simulink model "G59_LKAS_Carsim"  (R2018b)
settings: Solver=FixedStepDiscrete  StartTime=0.0  StopTime=30  FixedStep=0.001  RelTol=1e-3
InitFcn:
  | %{
  | delete_block('G59_LKAS_CarSim/LL');
  | delete_block('G59_LKAS_CarSim/LLClb');
  | path=cd('D:\Work\02_LKA\LKAS');
  | getFileName=ls(strcat(pwd,'\*.slx'));
  | filename = getFileName(1:4);
  | open_system(filename);
  | add_block('LKAS/LKAS/LL','G59_LKAS_CarSim/LL');
  | add_block('LKAS/LKAS/LLClb','G59_LKAS_CarSim/LLClb');
  | close_system(filename);
  | path=cd('D:\Program Files (x86)\CarSim2019.1_Data_LKA');
  | %}
model workspace (MAT data in the model file):
  LKA_CarWidth = Simulink.Parameter
  LKA_CarWidth.Value = 1.88
  LKA_CarWidth.DataType = 'single'
  LKA_CarWidth.Dimensions = [1 1]
  LKA_SampleTime = Simulink.Parameter
  LKA_SampleTime.Value = 0.001
  LKA_SampleTime.DataType = 'single'
  LKA_SampleTime.Dimensions = [1 1]
  LKA_StrRatio_C = Simulink.Parameter
  LKA_StrRatio_C.Value = 15.3
  LKA_StrRatio_C.DataType = 'single'
  LKA_StrRatio_C.Dimensions = [1 1]
  LKA_Veh2CamL_C = Simulink.Parameter
  LKA_Veh2CamL_C.Value = 3.68
  LKA_Veh2CamL_C.DataType = 'single'
  LKA_Veh2CamL_C.Dimensions = [1 1]
  LKA_Veh2CamW_C = Simulink.Parameter
  LKA_Veh2CamW_C.Value = 0.94
  LKA_Veh2CamW_C.DataType = 'single'
  LKA_Veh2CamW_C.Dimensions = [1 1]
  LKA_WhlBaseL_C = Simulink.Parameter
  LKA_WhlBaseL_C.Value = 2.8
  LKA_WhlBaseL_C.DataType = 'single'
  LKA_WhlBaseL_C.Dimensions = [1 1]
  LL_CompSWA_C = Simulink.Parameter
  LL_CompSWA_C.Value = 0
  LL_CompSWA_C.DataType = 'single'
  LL_CompSWA_C.Dimensions = [1 1]
  LL_CrvtPrvwT_C = Simulink.Parameter
  LL_CrvtPrvwT_C.Value = 0.45
  LL_CrvtPrvwT_C.DataType = 'single'
  LL_CrvtPrvwT_C.Dimensions = [1 1]
  LL_DesDvt_C = Simulink.Parameter
  LL_DesDvt_C.Value = 0.2
  LL_DesDvt_C.DataType = 'single'
  LL_DesDvt_C.Dimensions = [1 1]
  LL_DvtComp_C = Simulink.Parameter
  LL_DvtComp_C.Value = 0
  LL_DvtComp_C.DataType = 'single'
  LL_DvtComp_C.Dimensions = [1 1]
  LL_DvtPrvwT_C = Simulink.Parameter
  LL_DvtPrvwT_C.Value = 0.45
  LL_DvtPrvwT_C.DataType = 'single'
  LL_DvtPrvwT_C.Dimensions = [1 1]
  LL_DvtSpdDet_vDvtSpdMin_C = Simulink.Parameter
  LL_DvtSpdDet_vDvtSpdMin_C.Value = 0
  LL_DvtSpdDet_vDvtSpdMin_C.DataType = 'single'
  LL_DvtSpdDet_vDvtSpdMin_C.Dimensions = [1 1]
  LL_HdAgExT_C = Simulink.Parameter
  LL_HdAgExT_C.Value = 15
  LL_HdAgExT_C.DataType = 'single'
  LL_HdAgExT_C.Dimensions = [1 1]
  LL_HdAgPrvwT_C = Simulink.Parameter
  LL_HdAgPrvwT_C.Value = 0.45
  LL_HdAgPrvwT_C.DataType = 'single'
  LL_HdAgPrvwT_C.Dimensions = [1 1]
  LL_LAccMax_C = Simulink.Parameter
  LL_LAccMax_C.Value = 3
  LL_LAccMax_C.DataType = 'single'
  LL_LAccMax_C.Dimensions = [1 1]
  LL_LAccRMax_C = Simulink.Parameter
  LL_LAccRMax_C.Value = 5
  LL_LAccRMax_C.DataType = 'single'
  LL_LAccRMax_C.Dimensions = [1 1]
  LL_LDWS_SUPPRESS_HEADING = Simulink.Parameter
  LL_LDWS_SUPPRESS_HEADING.Value = 2
  LL_LDWS_SUPPRESS_HEADING.DataType = 'single'
  LL_LDWS_SUPPRESS_HEADING.Dimensions = [1 1]
  LL_LDW_EarliestWarnLine_C = Simulink.Parameter
  LL_LDW_EarliestWarnLine_C.Value = 0.3
  LL_LDW_EarliestWarnLine_C.DataType = 'single'
  LL_LDW_EarliestWarnLine_C.Dimensions = [1 1]
  LL_LDW_LatestWarnLine_C = Simulink.Parameter
  LL_LDW_LatestWarnLine_C.Value = -0.4
  LL_LDW_LatestWarnLine_C.DataType = 'single'
  LL_LDW_LatestWarnLine_C.Dimensions = [1 1]
  LL_LFClb_TFC_FfCtlRatio_C = Simulink.Parameter
  LL_LFClb_TFC_FfCtlRatio_C.Value = 1
  LL_LFClb_TFC_FfCtlRatio_C.DataType = 'single'
  LL_LFClb_TFC_FfCtlRatio_C.Dimensions = [1 1]
  LL_LFClb_TFC_KdBalance_C = Simulink.Parameter
  LL_LFClb_TFC_KdBalance_C.Value = 0
  LL_LFClb_TFC_KdBalance_C.DataType = 'single'
  LL_LFClb_TFC_KdBalance_C.Dimensions = [1 1]
  LL_LFClb_TFC_KdMaxSWA_C = Simulink.Parameter
  LL_LFClb_TFC_KdMaxSWA_C.Value = 20
  LL_LFClb_TFC_KdMaxSWA_C.DataType = 'single'
  LL_LFClb_TFC_KdMaxSWA_C.Dimensions = [1 1]
  LL_LFClb_TFC_KdV1_C = Simulink.Parameter
  LL_LFClb_TFC_KdV1_C.Value = 250
  LL_LFClb_TFC_KdV1_C.DataType = 'single'
  LL_LFClb_TFC_KdV1_C.Dimensions = [1 1]
  LL_LFClb_TFC_KdV2_C = Simulink.Parameter
  LL_LFClb_TFC_KdV2_C.Value = 250
  LL_LFClb_TFC_KdV2_C.DataType = 'single'
  LL_LFClb_TFC_KdV2_C.Dimensions = [1 1]
  LL_LFClb_TFC_KdVehSpdLwr_C = Simulink.Parameter
  LL_LFClb_TFC_KdVehSpdLwr_C.Value = 60
  LL_LFClb_TFC_KdVehSpdLwr_C.DataType = 'single'
  LL_LFClb_TFC_KdVehSpdLwr_C.Dimensions = [1 1]
  LL_LFClb_TFC_KdVehSpdUpr_C = Simulink.Parameter
  LL_LFClb_TFC_KdVehSpdUpr_C.Value = 120
  LL_LFClb_TFC_KdVehSpdUpr_C.DataType = 'single'
  LL_LFClb_TFC_KdVehSpdUpr_C.Dimensions = [1 1]
  LL_LFClb_TFC_KiMaxSWA_C = Simulink.Parameter
  LL_LFClb_TFC_KiMaxSWA_C.Value = 5
  LL_LFClb_TFC_KiMaxSWA_C.DataType = 'single'
  LL_LFClb_TFC_KiMaxSWA_C.Dimensions = [1 1]
  LL_LFClb_TFC_Ki_C = Simulink.Parameter
  LL_LFClb_TFC_Ki_C.Value = 0.002
  LL_LFClb_TFC_Ki_C.DataType = 'single'
  LL_LFClb_TFC_Ki_C.Dimensions = [1 1]
  LL_LFClb_TFC_KpKlat_C = Simulink.Parameter
  LL_LFClb_TFC_KpKlat_C.Value = -4.5
  LL_LFClb_TFC_KpKlat_C.DataType = 'single'
  LL_LFClb_TFC_KpKlat_C.Dimensions = [1 1]
  LL_LFClb_TFC_KpV1_C = Simulink.Parameter
  LL_LFClb_TFC_KpV1_C.Value = 40
  LL_LFClb_TFC_KpV1_C.DataType = 'single'
  LL_LFClb_TFC_KpV1_C.Dimensions = [1 1]
  LL_LFClb_TFC_KpV2_C = Simulink.Parameter
  LL_LFClb_TFC_KpV2_C.Value = 40
  LL_LFClb_TFC_KpV2_C.DataType = 'single'
  LL_LFClb_TFC_KpV2_C.Dimensions = [1 1]
  LL_LFClb_TFC_KpVehSpdLwr_C = Simulink.Parameter
  LL_LFClb_TFC_KpVehSpdLwr_C.Value = 60
  LL_LFClb_TFC_KpVehSpdLwr_C.DataType = 'single'
  LL_LFClb_TFC_KpVehSpdLwr_C.Dimensions = [1 1]
  LL_LFClb_TFC_KpVehSpdUpr_C = Simulink.Parameter
  LL_LFClb_TFC_KpVehSpdUpr_C.Value = 120
  LL_LFClb_TFC_KpVehSpdUpr_C.DataType = 'single'
  LL_LFClb_TFC_KpVehSpdUpr_C.Dimensions = [1 1]
  LL_LFClb_TFC_Kp_C = Simulink.Parameter
  LL_LFClb_TFC_Kp_C.Value = 1
  LL_LFClb_TFC_Kp_C.DataType = 'single'
  LL_LFClb_TFC_Kp_C.Dimensions = [1 1]
  LL_LFClb_TFC_PrvwT_C = Simulink.Parameter
  LL_LFClb_TFC_PrvwT_C.Value = 2
  LL_LFClb_TFC_PrvwT_C.DataType = 'single'
  LL_LFClb_TFC_PrvwT_C.Dimensions = [1 1]
  LL_LKAExPrcs_ExitC0Dvt = Simulink.Parameter
  LL_LKAExPrcs_ExitC0Dvt.Value = 0.01
  LL_LKAExPrcs_ExitC0Dvt.DataType = 'single'
  LL_LKAExPrcs_ExitC0Dvt.Dimensions = [1 1]
  LL_LKAExPrcs_ExitC0Swt = Simulink.Parameter
  LL_LKAExPrcs_ExitC0Swt.Value = 1
  LL_LKAExPrcs_ExitC0Swt.DataType = 'boolean'
  LL_LKAExPrcs_ExitC0Swt.Dimensions = [1 1]
  LL_LKAExPrcs_tiExitTime1 = Simulink.Parameter
  LL_LKAExPrcs_tiExitTime1.Value = 8
  LL_LKAExPrcs_tiExitTime1.DataType = 'single'
  LL_LKAExPrcs_tiExitTime1.Dimensions = [1 1]
  LL_LKAExPrcs_tiExitTime2 = Simulink.Parameter
  LL_LKAExPrcs_tiExitTime2.Value = 4
  LL_LKAExPrcs_tiExitTime2.DataType = 'single'
  LL_LKAExPrcs_tiExitTime2.Dimensions = [1 1]
  LL_LKAExPrcs_tiExitTime3 = Simulink.Parameter
  LL_LKAExPrcs_tiExitTime3.Value = 0.2
  LL_LKAExPrcs_tiExitTime3.DataType = 'single'
  LL_LKAExPrcs_tiExitTime3.Dimensions = [1 1]
  LL_LKASWASyn_M0 = Simulink.Parameter
  LL_LKASWASyn_M0.Value = 0.4
  LL_LKASWASyn_M0.DataType = 'single'
  LL_LKASWASyn_M0.Dimensions = [1 1]
  LL_LKASWASyn_M1 = Simulink.Parameter
  LL_LKASWASyn_M1.Value = 0.8
  LL_LKASWASyn_M1.DataType = 'single'
  LL_LKASWASyn_M1.Dimensions = [1 1]
  LL_LKASWASyn_M2 = Simulink.Parameter
  LL_LKASWASyn_M2.Value = 0.3
  LL_LKASWASyn_M2.DataType = 'single'
  LL_LKASWASyn_M2.Dimensions = [1 1]
  LL_LKASWASyn_M3K = Simulink.Parameter
  LL_LKASWASyn_M3K.Value = 0.2
  LL_LKASWASyn_M3K.DataType = 'single'
  LL_LKASWASyn_M3K.Dimensions = [1 1]
  LL_LKASWASyn_SWAaddMax = Simulink.Parameter
  LL_LKASWASyn_SWAaddMax.Value = 8
  LL_LKASWASyn_SWAaddMax.DataType = 'single'
  LL_LKASWASyn_SWAaddMax.Dimensions = [1 1]
  LL_LKASWASyn_T2 = Simulink.Parameter
  LL_LKASWASyn_T2.Value = 4
  LL_LKASWASyn_T2.DataType = 'single'
  LL_LKASWASyn_T2.Dimensions = [1 1]
  LL_LKASWASyn_TrqMax = Simulink.Parameter
  LL_LKASWASyn_TrqMax.Value = 1.5
  LL_LKASWASyn_TrqMax.DataType = 'single'
  LL_LKASWASyn_TrqMax.Dimensions = [1 1]
  LL_LKASWASyn_TrqSwaAddSwt = Simulink.Parameter
  LL_LKASWASyn_TrqSwaAddSwt.Value = 0
  LL_LKASWASyn_TrqSwaAddSwt.DataType = 'boolean'
  LL_LKASWASyn_TrqSwaAddSwt.Dimensions = [1 1]
  LL_LKASWASyn_TrqSwaRateDiff = Simulink.Parameter
  LL_LKASWASyn_TrqSwaRateDiff.Value = -0.2
  LL_LKASWASyn_TrqSwaRateDiff.DataType = 'single'
  LL_LKASWASyn_TrqSwaRateDiff.Dimensions = [1 1]
  LL_LKASWASyn_tiTrqSwaRtTime = Simulink.Parameter
  LL_LKASWASyn_tiTrqSwaRtTime.Value = 0.2
  LL_LKASWASyn_tiTrqSwaRtTime.DataType = 'single'
  LL_LKASWASyn_tiTrqSwaRtTime.Dimensions = [1 1]
  LL_LKASWASyn_tiTrqSwaTime = Simulink.Parameter
  LL_LKASWASyn_tiTrqSwaTime.Value = 0.3
  LL_LKASWASyn_tiTrqSwaTime.DataType = 'single'
  LL_LKASWASyn_tiTrqSwaTime.Dimensions = [1 1]
  LL_LKAS_OUT_OF_CONTROL_LAT_VEL = Simulink.Parameter
  LL_LKAS_OUT_OF_CONTROL_LAT_VEL.Value = 1.5
  LL_LKAS_OUT_OF_CONTROL_LAT_VEL.DataType = 'single'
  LL_LKAS_OUT_OF_CONTROL_LAT_VEL.Dimensions = [1 1]
  LL_LKAS_OUT_OF_CONTROL_TTLC = Simulink.Parameter
  LL_LKAS_OUT_OF_CONTROL_TTLC.Value = 0.3
  LL_LKAS_OUT_OF_CONTROL_TTLC.DataType = 'single'
  LL_LKAS_OUT_OF_CONTROL_TTLC.Dimensions = [1 1]
  LL_LKA_EarliestWarnLine_C = Simulink.Parameter
  LL_LKA_EarliestWarnLine_C.Value = 0.3
  LL_LKA_EarliestWarnLine_C.DataType = 'single'
  LL_LKA_EarliestWarnLine_C.Dimensions = [1 1]
  LL_LKA_LatestWarnLine_C = Simulink.Parameter
  LL_LKA_LatestWarnLine_C.Value = -0.5
  LL_LKA_LatestWarnLine_C.DataType = 'single'
  LL_LKA_LatestWarnLine_C.Dimensions = [1 1]
  LL_LSpdCompT_C = Simulink.Parameter
  LL_LSpdCompT_C.Value = 0.4
  LL_LSpdCompT_C.DataType = 'single'
  LL_LSpdCompT_C.Dimensions = [1 1]
  LL_LaneSelect = Simulink.Parameter
  LL_LaneSelect.Value = 1
  LL_LaneSelect.DataType = 'single'
  LL_LaneSelect.Dimensions = [1 1]
  LL_MAX_DELAY_EPSSTAR_TIME = Simulink.Parameter
  LL_MAX_DELAY_EPSSTAR_TIME.Value = 0.5
  LL_MAX_DELAY_EPSSTAR_TIME.DataType = 'single'
  LL_MAX_DELAY_EPSSTAR_TIME.Dimensions = [1 1]
  LL_MAX_DRIVER_TORQUE_DISABLE = Simulink.Parameter
  LL_MAX_DRIVER_TORQUE_DISABLE.Value = 2.25
  LL_MAX_DRIVER_TORQUE_DISABLE.DataType = 'single'
  LL_MAX_DRIVER_TORQUE_DISABLE.Dimensions = [1 1]
  LL_MAX_DRIVER_TORQUE_ENABLE = Simulink.Parameter
  LL_MAX_DRIVER_TORQUE_ENABLE.Value = 3
  LL_MAX_DRIVER_TORQUE_ENABLE.DataType = 'single'
  LL_MAX_DRIVER_TORQUE_ENABLE.Dimensions = [1 1]
  LL_MAX_LANE_WIDTH_DISABLE = Simulink.Parameter
  LL_MAX_LANE_WIDTH_DISABLE.Value = 5.5
  LL_MAX_LANE_WIDTH_DISABLE.DataType = 'single'
  LL_MAX_LANE_WIDTH_DISABLE.Dimensions = [1 1]
  LL_MAX_LANE_WIDTH_ENABLE = Simulink.Parameter
  LL_MAX_LANE_WIDTH_ENABLE.Value = 5.4
  LL_MAX_LANE_WIDTH_ENABLE.DataType = 'single'
  LL_MAX_LANE_WIDTH_ENABLE.Dimensions = [1 1]
  LL_MAX_LAT_ACC_DISABLE = Simulink.Parameter
  LL_MAX_LAT_ACC_DISABLE.Value = 3.5
  LL_MAX_LAT_ACC_DISABLE.DataType = 'single'
  LL_MAX_LAT_ACC_DISABLE.Dimensions = [1 1]
  LL_MAX_LAT_ACC_ENABLE = Simulink.Parameter
  LL_MAX_LAT_ACC_ENABLE.Value = 3
  LL_MAX_LAT_ACC_ENABLE.DataType = 'single'
  LL_MAX_LAT_ACC_ENABLE.Dimensions = [1 1]
  LL_MAX_LDWS_SPEED_DISABLE = Simulink.Parameter
  LL_MAX_LDWS_SPEED_DISABLE.Value = 150
  LL_MAX_LDWS_SPEED_DISABLE.DataType = 'single'
  LL_MAX_LDWS_SPEED_DISABLE.Dimensions = [1 1]
  LL_MAX_LDWS_SPEED_ENABLE = Simulink.Parameter
  LL_MAX_LDWS_SPEED_ENABLE.Value = 140
  LL_MAX_LDWS_SPEED_ENABLE.DataType = 'single'
  LL_MAX_LDWS_SPEED_ENABLE.Dimensions = [1 1]
  LL_MAX_LKAS_SPEED_DISABLE = Simulink.Parameter
  LL_MAX_LKAS_SPEED_DISABLE.Value = 150
  LL_MAX_LKAS_SPEED_DISABLE.DataType = 'single'
  LL_MAX_LKAS_SPEED_DISABLE.Dimensions = [1 1]
  LL_MAX_LKAS_SPEED_ENABLE = Simulink.Parameter
  LL_MAX_LKAS_SPEED_ENABLE.Value = 140
  LL_MAX_LKAS_SPEED_ENABLE.DataType = 'single'
  LL_MAX_LKAS_SPEED_ENABLE.Dimensions = [1 1]
  LL_MAX_LONG_ACC_DISABLE = Simulink.Parameter
  LL_MAX_LONG_ACC_DISABLE.Value = 3.5
  LL_MAX_LONG_ACC_DISABLE.DataType = 'single'
  LL_MAX_LONG_ACC_DISABLE.Dimensions = [1 1]
  LL_MAX_LONG_ACC_ENABLE = Simulink.Parameter
  LL_MAX_LONG_ACC_ENABLE.Value = 3
  LL_MAX_LONG_ACC_ENABLE.DataType = 'single'
  LL_MAX_LONG_ACC_ENABLE.Dimensions = [1 1]
  LL_MAX_LONG_DECEL_DISABLE = Simulink.Parameter
  LL_MAX_LONG_DECEL_DISABLE.Value = 2.5
  LL_MAX_LONG_DECEL_DISABLE.DataType = 'single'
  LL_MAX_LONG_DECEL_DISABLE.Dimensions = [1 1]
  LL_MAX_LONG_DECEL_ENABLE = Simulink.Parameter
  LL_MAX_LONG_DECEL_ENABLE.Value = 2
  LL_MAX_LONG_DECEL_ENABLE.DataType = 'single'
  LL_MAX_LONG_DECEL_ENABLE.Dimensions = [1 1]
  LL_MAX_STEER_ANGLE_DISABLE = Simulink.Parameter
  LL_MAX_STEER_ANGLE_DISABLE.Value = 70
  LL_MAX_STEER_ANGLE_DISABLE.DataType = 'single'
  LL_MAX_STEER_ANGLE_DISABLE.Dimensions = [1 1]
  LL_MAX_STEER_ANGLE_ENABLE = Simulink.Parameter
  LL_MAX_STEER_ANGLE_ENABLE.Value = 60
  LL_MAX_STEER_ANGLE_ENABLE.DataType = 'single'
  LL_MAX_STEER_ANGLE_ENABLE.Dimensions = [1 1]
  LL_MAX_STEER_SPEED_DISABLE = Simulink.Parameter
  LL_MAX_STEER_SPEED_DISABLE.Value = 5000
  LL_MAX_STEER_SPEED_DISABLE.DataType = 'single'
  LL_MAX_STEER_SPEED_DISABLE.Dimensions = [1 1]
  LL_MAX_STEER_SPEED_ENABLE = Simulink.Parameter
  LL_MAX_STEER_SPEED_ENABLE.Value = 5000
  LL_MAX_STEER_SPEED_ENABLE.DataType = 'single'
  LL_MAX_STEER_SPEED_ENABLE.Dimensions = [1 1]
  LL_MAX_SYSTEM_CURVATURE_DISABLE = Simulink.Parameter
  LL_MAX_SYSTEM_CURVATURE_DISABLE.Value = 0.005
  LL_MAX_SYSTEM_CURVATURE_DISABLE.DataType = 'single'
  LL_MAX_SYSTEM_CURVATURE_DISABLE.Dimensions = [1 1]
  LL_MAX_SYSTEM_CURVATURE_ENABLE = Simulink.Parameter
  LL_MAX_SYSTEM_CURVATURE_ENABLE.Value = 0.004
  LL_MAX_SYSTEM_CURVATURE_ENABLE.DataType = 'single'
  LL_MAX_SYSTEM_CURVATURE_ENABLE.Dimensions = [1 1]
  LL_MIN_LANE_WIDTH_DISABLE = Simulink.Parameter
  LL_MIN_LANE_WIDTH_DISABLE.Value = 2.4
  LL_MIN_LANE_WIDTH_DISABLE.DataType = 'single'
  LL_MIN_LANE_WIDTH_DISABLE.Dimensions = [1 1]
  LL_MIN_LANE_WIDTH_ENABLE = Simulink.Parameter
  LL_MIN_LANE_WIDTH_ENABLE.Value = 2.5
  LL_MIN_LANE_WIDTH_ENABLE.DataType = 'single'
  LL_MIN_LANE_WIDTH_ENABLE.Dimensions = [1 1]
  LL_MIN_LKAS_SPEED_DISABLE = Simulink.Parameter
  LL_MIN_LKAS_SPEED_DISABLE.Value = 55
  LL_MIN_LKAS_SPEED_DISABLE.DataType = 'single'
  LL_MIN_LKAS_SPEED_DISABLE.Dimensions = [1 1]
  LL_MIN_LKAS_SPEED_ENABLE = Simulink.Parameter
  LL_MIN_LKAS_SPEED_ENABLE.Value = 60
  LL_MIN_LKAS_SPEED_ENABLE.DataType = 'single'
  LL_MIN_LKAS_SPEED_ENABLE.Dimensions = [1 1]
  LL_Max_LDWS_Warning_Time = Simulink.Parameter
  LL_Max_LDWS_Warning_Time.Value = 5
  LL_Max_LDWS_Warning_Time.DataType = 'single'
  LL_Max_LDWS_Warning_Time.Dimensions = [1 1]
  LL_NomTAhd_C = Simulink.Parameter
  LL_NomTAhd_C.Value = 0.2
  LL_NomTAhd_C.DataType = 'single'
  LL_NomTAhd_C.Dimensions = [1 1]
  LL_RlsDet_tiTDelTime_DISABLE = Simulink.Parameter
  LL_RlsDet_tiTDelTime_DISABLE.Value = 20
  LL_RlsDet_tiTDelTime_DISABLE.DataType = 'single'
  LL_RlsDet_tiTDelTime_DISABLE.Dimensions = [1 1]
  LL_RlsDet_tiTrqChkT_DISABLE = Simulink.Parameter
  LL_RlsDet_tiTrqChkT_DISABLE.Value = 0.25
  LL_RlsDet_tiTrqChkT_DISABLE.DataType = 'single'
  LL_RlsDet_tiTrqChkT_DISABLE.Dimensions = [1 1]
  LL_RlsDet_tiTrqChkT_EPS_DISABLE = Simulink.Parameter
  LL_RlsDet_tiTrqChkT_EPS_DISABLE.Value = 0.5
  LL_RlsDet_tiTrqChkT_EPS_DISABLE.DataType = 'single'
  LL_RlsDet_tiTrqChkT_EPS_DISABLE.Dimensions = [1 1]
  LL_ThresDet_lDvtThresLwrLDW = Simulink.Parameter
  LL_ThresDet_lDvtThresLwrLDW.Value = 0.15
  LL_ThresDet_lDvtThresLwrLDW.DataType = 'single'
  LL_ThresDet_lDvtThresLwrLDW.Dimensions = [1 1]
  LL_ThresDet_lDvtThresLwrLKA = Simulink.Parameter
  LL_ThresDet_lDvtThresLwrLKA.Value = 0.3
  LL_ThresDet_lDvtThresLwrLKA.DataType = 'single'
  LL_ThresDet_lDvtThresLwrLKA.Dimensions = [1 1]
  LL_ThresDet_lDvtThresUprLDW = Simulink.Parameter
  LL_ThresDet_lDvtThresUprLDW.Value = 0.3
  LL_ThresDet_lDvtThresUprLDW.DataType = 'single'
  LL_ThresDet_lDvtThresUprLDW.Dimensions = [1 1]
  LL_ThresDet_lDvtThresUprLKA = Simulink.Parameter
  LL_ThresDet_lDvtThresUprLKA.Value = 0.6
  LL_ThresDet_lDvtThresUprLKA.DataType = 'single'
  LL_ThresDet_lDvtThresUprLKA.Dimensions = [1 1]
  LL_ThresDet_tiTTLCThresLDW = Simulink.Parameter
  LL_ThresDet_tiTTLCThresLDW.Value = 0.75
  LL_ThresDet_tiTTLCThresLDW.DataType = 'single'
  LL_ThresDet_tiTTLCThresLDW.Dimensions = [1 1]
  LL_ThresDet_tiTTLCThresLKA = Simulink.Parameter
  LL_ThresDet_tiTTLCThresLKA.Value = 1.5
  LL_ThresDet_tiTTLCThresLKA.DataType = 'single'
  LL_ThresDet_tiTTLCThresLKA.Dimensions = [1 1]
  LL_TkOvStChk_tiTDelTime = Simulink.Parameter
  LL_TkOvStChk_tiTDelTime.Value = 2
  LL_TkOvStChk_tiTDelTime.DataType = 'single'
  LL_TkOvStChk_tiTDelTime.Dimensions = [1 1]
  LL_TkOvStChk_tiTDelTime_DEACTV = Simulink.Parameter
  LL_TkOvStChk_tiTDelTime_DEACTV.Value = 1
  LL_TkOvStChk_tiTDelTime_DEACTV.DataType = 'single'
  LL_TkOvStChk_tiTDelTime_DEACTV.Dimensions = [1 1]
  LL_TkOvStChk_tiTrqChkT = Simulink.Parameter
  LL_TkOvStChk_tiTrqChkT.Value = 0.1
  LL_TkOvStChk_tiTrqChkT.DataType = 'single'
  LL_TkOvStChk_tiTrqChkT.Dimensions = [1 1]
  LL_TkOvStChk_tiTrqChkT_DEACTV = Simulink.Parameter
  LL_TkOvStChk_tiTrqChkT_DEACTV.Value = 0.2
  LL_TkOvStChk_tiTrqChkT_DEACTV.DataType = 'single'
  LL_TkOvStChk_tiTrqChkT_DEACTV.Dimensions = [1 1]
  LL_lStpLngth_C = Simulink.Parameter
  LL_lStpLngth_C.Value = 5
  LL_lStpLngth_C.DataType = 'single'
  LL_lStpLngth_C.Dimensions = [1 1]
  ob_LKA_Disable_Reason = Simulink.Signal
  ob_LKA_Disable_Reason.DataType = 'single'
  ob_LKA_Disable_Reason.Dimensions = -1
  ob_LKA_Disable_Reason.DimensionsMode = 'auto'
  ob_LKA_Disable_Reason.Complexity = 'auto'
  ob_LKA_Disable_Reason.SampleTime = -1
  ob_LKA_Disable_Reason.SamplingMode = 'auto'
  ob_LKA_LKADeactvCSyn = Simulink.Signal
  ob_LKA_LKADeactvCSyn.DataType = 'single'
  ob_LKA_LKADeactvCSyn.Dimensions = -1
  ob_LKA_LKADeactvCSyn.DimensionsMode = 'auto'
  ob_LKA_LKADeactvCSyn.Complexity = 'auto'
  ob_LKA_LKADeactvCSyn.SampleTime = -1
  ob_LKA_LKADeactvCSyn.SamplingMode = 'auto'
  ob_LKA_Version = Simulink.Signal
  ob_LKA_Version.DataType = 'single'
  ob_LKA_Version.Dimensions = -1
  ob_LKA_Version.DimensionsMode = 'auto'
  ob_LKA_Version.Complexity = 'auto'
  ob_LKA_Version.SampleTime = -1
  ob_LKA_Version.SamplingMode = 'auto'
undefined symbols (not defined in the file): LKA_CarWidth, LKA_SampleTime, LKA_StrRatio_C, LKA_Veh2CamL_C, LKA_Veh2CamW_C, LKA_WhlBaseL_C, LL_CompSWA_C, LL_CrvtPrvwT_C, LL_DesDvt_C, LL_DvtComp_C, LL_DvtPrvwT_C, LL_DvtSpdDet_vDvtSpdMin_C, LL_HdAgExT_C, LL_HdAgPrvwT_C, LL_LAccMax_C, LL_LAccRMax_C, LL_LDW_EarliestWarnLine_C, LL_LDW_LatestWarnLine_C, LL_LDWS_SUPPRESS_HEADING, LL_LFClb_TFC_FfCtlRatio_C, LL_LFClb_TFC_KdBalance_C, LL_LFClb_TFC_KdMaxSWA_C, LL_LFClb_TFC_KdV1_C, LL_LFClb_TFC_KdV2_C, LL_LFClb_TFC_KdVehSpdLwr_C, LL_LFClb_TFC_KdVehSpdUpr_C, LL_LFClb_TFC_Ki_C, LL_LFClb_TFC_KiMaxSWA_C, LL_LFClb_TFC_Kp_C, LL_LFClb_TFC_KpKlat_C, LL_LFClb_TFC_KpV1_C, LL_LFClb_TFC_KpV2_C, LL_LFClb_TFC_KpVehSpdLwr_C, LL_LFClb_TFC_KpVehSpdUpr_C, LL_LFClb_TFC_PrvwT_C, LL_LKA_EarliestWarnLine_C, LL_LKA_LatestWarnLine_C, LL_LKAExPrcs_ExitC0Dvt, LL_LKAExPrcs_ExitC0Swt, LL_LKAExPrcs_tiExitTime1, LL_LKAExPrcs_tiExitTime2, LL_LKAExPrcs_tiExitTime3, LL_LKAS_OUT_OF_CONTROL_LAT_VEL, LL_LKAS_OUT_OF_CONTROL_TTLC, LL_LKASWASyn_M0, LL_LKASWASyn_M1, LL_LKASWASyn_M2, LL_LKASWASyn_M3K, LL_LKASWASyn_SWAaddMax, LL_LKASWASyn_T2, LL_LKASWASyn_tiTrqSwaRtTime, LL_LKASWASyn_tiTrqSwaTime, LL_LKASWASyn_TrqMax, LL_LKASWASyn_TrqSwaAddSwt, LL_LKASWASyn_TrqSwaRateDiff, LL_LSpdCompT_C, LL_lStpLngth_C, LL_MAX_DELAY_EPSSTAR_TIME, LL_MAX_DRIVER_TORQUE_DISABLE, LL_MAX_DRIVER_TORQUE_ENABLE ... (+38)
libraries: simulink x138, dspstat3 x3, Solver_SF x1, simulink_extras x1
(part 1 of 13)
settings Model: PauseTimes=15.416  Creator=ADMIN  LastModifiedBy=hejr
settings DebuggingCC: UnderspecifiedInitializationDetection=Classic  ParameterOverflowMsg=none

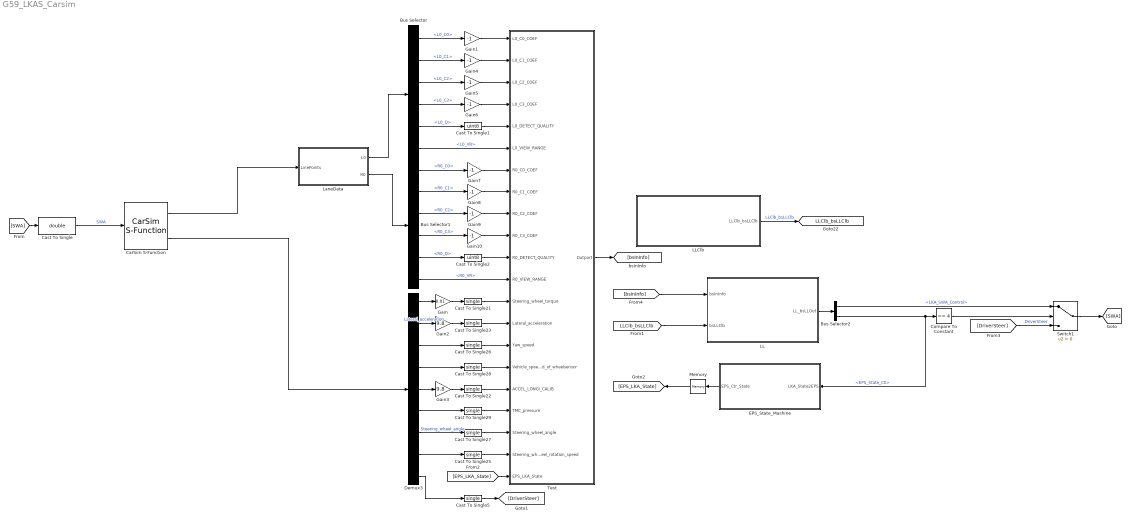
== system G59_LKAS_Carsim ==
  Bus Selector : BusSelector  OutputSignals=L0_C0,L0_C1,L0_C2,L0_C3,L0_Q,L0_VR
  Bus Selector1 : BusSelector  OutputSignals=R0_C0,R0_C1,R0_C2,R0_C3,R0_Q,R0_VR
  Bus Selector2 : BusSelector  OutputSignals=LKA_SWA_Control,EPS_State_Ctl
  CarSim S-Function : Solver_SF/CarSim S-Function  Priority=1  SIMFILE=simfile.sim  Run_RTs=off  vs_state_ind=Run  StopMode_ind=Vehicle Model
  Cast To Single : DataTypeConversion  OutDataTypeStr=double
  Cast To Single1 : DataTypeConversion  OutDataTypeStr=uint8
  Cast To Single2 : DataTypeConversion  OutDataTypeStr=uint8
  Cast To Single{5,21..23,25..29} (9 alike) : DataTypeConversion  OutDataTypeStr=single
  Compare To Constant : simulink/Logic and Bit Operations/Compare To Constant  relop===  const=4  OutDataTypeStr=boolean
  Demux3 : Demux  Outputs=9
  EPS_State_Mashine : Subsystem
  Gain : Gain  Gain=0.01
  Gain{1,4..10} (8 alike) : Gain  Gain=-1
  Gain2 : Gain  Gain=9.8
  Gain3 : Gain  Gain=9.8
  LL : Subsystem
  LLClb : Subsystem
  LaneData : Subsystem
  Memory : Memory  InheritSampleTime=on
  Switch1 : Switch  Criteria=u2 > Threshold
  Test : Subsystem
  tag scope: LLClb_bsLLClb=global
  wires:
  Bus Selector1/1 -> Gain7/1  "<R0_C0>"
  Demux3/1 -> Gain/1
  Cast To Single1/1 -> Test/5(L0_DETECT_QUALITY)
  Cast To Single2/1 -> Test/11(R0_DETECT_QUALITY)
  Cast To Single21/1 -> Test/13(Steering_wheel_torque)
  Cast To Single27/1 -> Test/19(Steering_wheel_angle)
  Cast To Single23/1 -> Test/14(Lateral_acceleration)
  Cast To Single28/1 -> Test/16(Vehicle_speed_of_wheelsensor)
  Bus Selector/1 -> Gain1/1  "<L0_C0>"
  Bus Selector1/5 -> Cast To Single2/1  "<R0_Q>"
  [SWA] -> Cast To Single/1
  Cast To Single22/1 -> Test/17(ACCEL_LONGI_CALIB)
  Cast To Single29/1 -> Test/18(TMC_pressure)
  Bus Selector1/6 -> Test/12(R0_VIEW_RANGE)  "<R0_VR>"
  Cast To Single26/1 -> Test/15(Yaw_speed)
  Cast To Single/1 -> CarSim S-Function/1  "SWA"
  Bus Selector/5 -> Cast To Single1/1  "<L0_Q>"
  Bus Selector/2 -> Gain4/1  "<L0_C1>"
  Bus Selector/6 -> Test/6(L0_VIEW_RANGE)  "<L0_VR>"
  Bus Selector/4 -> Gain6/1  "<L0_C3>"
  Demux3/2 -> Gain2/1  "Lateral_acceleration"
  Demux3/8 -> Cast To Single25/1
  Bus Selector1/3 -> Gain9/1  "<R0_C2>"
  Demux3/6 -> Cast To Single29/1
  Demux3/3 -> Cast To Single26/1
  Bus Selector1/2 -> Gain8/1  "<R0_C1>"
  Demux3/7 -> Cast To Single27/1  "Steering_wheel_angle"
  Demux3/5 -> Gain3/1
  Demux3/4 -> Cast To Single28/1
  Bus Selector/3 -> Gain5/1  "<L0_C2>"
  Cast To Single25/1 -> Test/20(Steering_wheel_rotation_speed)
  Bus Selector1/4 -> Gain10/1  "<R0_C3>"
  LLClb/1(LLClb_bsLLClb) -> [LLClb_bsLLClb]  "LLClb_bsLLClb"
  [LLClb_bsLLClb] -> LL/2(bsLLClb)
  Bus Selector2/2 -> EPS_State_Mashine/1(LKA_State2EPS), Compare To Constant/1  "<EPS_State_Ctl>"
  EPS_State_Mashine/1(EPS_Ctr_State) -> Memory/1
  [bsInInfo] -> LL/1(bsInInfo)
  Gain/1 -> Cast To Single21/1
  LaneData/2(R0) -> Bus Selector1/1
  LaneData/1(L0) -> Bus Selector/1
  Bus Selector2/1 -> Switch1/1  "<LKA_SWA_Control>"
  Demux3/9 -> Cast To Single5/1
  Compare To Constant/1 -> Switch1/2
  [DriverSteer] -> Switch1/3  "DriverSteer"
  Switch1/1 -> [SWA]
  Cast To Single5/1 -> [DriverSteer]
  CarSim S-Function/1 -> LaneData/1(LinePoints)
  Gain2/1 -> Cast To Single23/1
  Gain3/1 -> Cast To Single22/1
  Test/1(Outport) -> [bsInInfo]
  Memory/1 -> [EPS_LKA_State]
  [EPS_LKA_State] -> Test/21(EPS_LKA_State)
  LL/1(LL_bsLLOut) -> Bus Selector2/1
  Gain1/1 -> Test/1(L0_C0_COEF)
  Gain4/1 -> Test/2(L0_C1_COEF)
  Gain5/1 -> Test/3(L0_C2_COEF)
  Gain6/1 -> Test/4(L0_C3_COEF)
  Gain7/1 -> Test/7(R0_C0_COEF)
  Gain8/1 -> Test/8(R0_C1_COEF)
  Gain9/1 -> Test/9(R0_C2_COEF)
  Gain10/1 -> Test/10(R0_C3_COEF)
  CarSim S-Function/2 -> Demux3/1

== system G59_LKAS_Carsim/EPS_State_Mashine ==
  LKA_State2EPS : Inport
  Data Type Conversion2 : DataTypeConversion  OutDataTypeStr=uint16
  Steering Angle Cmd Synthesis State Machine (SWASynSM) : Stateflow chart  TreatAsAtomicUnit=on
  EPS_Ctr_State : Outport
  wires:
  LKA_State2EPS/1 -> Data Type Conversion2/1
  Steering Angle Cmd Synthesis State Machine (SWASynSM)/1(EPS_Ctr_State) -> EPS_Ctr_State/1
  Data Type Conversion2/1 -> Steering Angle Cmd Synthesis State Machine (SWASynSM)/1(LKA_State2EPS)

== system G59_LKAS_Carsim/LL ==
  bsInInfo : Inport
  bsLLClb : Inport  Port=2
  Bus Selector : BusSelector  OutputSignals=bsMP5Info.LKA_Mode
  Bus Selector1 : BusSelector  OutputSignals=bsLaneInfo.bsR0Info.R0_Q,bsLaneInfo.bsL0Info.L0_Q
  Bus Selector2 : BusSelector  OutputSignals=bsEPSInfo
  Bus Selector3 : BusSelector  OutputSignals=LKA_State,LDW_State
  Bus Selector4 : BusSelector  OutputSignals=bsLaneInfo.Fusion_AdditionalInf.Carema_Status
  Bus Selector5 : BusSelector  OutputSignals=bsMP5Info.LKA_Mode
  Fault_Diagnostic : Subsystem
  Ground1 : Ground
  Ground3 : Ground
  Human Machine Interface (HMI) : Subsystem
  LL Inputs Mapping : Subsystem
  LLOn : Subsystem
  LLOut : Subsystem
  Terminator : Terminator
  Version : Constant  Value=211105  OutMin=20410  OutMax=220630  OutDataTypeStr=single
  LL_bsLLOut : Outport
      settings: AttributesFormatString=Disable Action: %<OutputWhenDisabled>
  tag scope: LLMon=global
  wires:
  [bsSignalFault] -> LLOn/3(bsSignalFault)
  [bsLLClb] -> LLOn/2(bsLLClb)
  [bsInfo] -> LLOn/1(bsInInfo), Bus Selector/1
  [bsInInfo] -> LL Inputs Mapping/1(bsInInfo)
  LL Inputs Mapping/1(bsInfo) -> [bsInfo]
  [bsInInfo] -> Fault_Diagnostic/1(bsInInfo)
  Fault_Diagnostic/1(bsSignalFault) -> [bsSignalFault]
  LLOn/5(LLMon) -> [LLMon]
  LLOn/4(M) -> [LLOn_M]
  LLOn/3(phiSWACmd) -> [LLOn_phiSWACmd]
  LLOn/1(bsLLState) -> [LLOn_bsLLState]
  bsLLClb/1 -> [bsLLClb]
  LLOn/2(LDW_Flag) -> [LLOn_bsLDWWarnInfo]
  Version/1 -> Terminator/1  "ob_LKA_Version"
  Human Machine Interface (HMI)/1(HMI_LDWLKA) -> [HMI_bsLLHMI]  "bsLLHMI"
  bsInInfo/1 -> [bsInInfo]
  Bus Selector/1 -> LLOn/Enable  "<LKA_Mode>"
  [HMI_bsLLHMI] -> LLOut/3(LLOut_bsLLHMI)
  LLOut/1(LL_bsLLOut) -> LL_bsLLOut/1
  [LLOn_bsLLState] -> LLOut/1(LLOut_bsLLState)
  [LLOn_M] -> LLOut/4(LLOut_M)
  [bsInfo] -> LLOut/5(LLOut_bsInfo)
  [LLOn_phiSWACmd] -> LLOut/2(LLOut_phiSWACmd)
  [bsInfo] -> Bus Selector4/1, Bus Selector2/1, Bus Selector1/1, Bus Selector5/1
  Bus Selector3/2 -> Human Machine Interface (HMI)/3(HMI_LDW_STATE)  "<LDW_State>"
  Bus Selector3/1 -> Human Machine Interface (HMI)/2(HMI_LKA_STATE)  "<LKA_State>"
  Ground3/1 -> Human Machine Interface (HMI)/10(HMI_stFaultCSyn)
  Ground1/1 -> Human Machine Interface (HMI)/8(HMI_camera_common_fault)
  Bus Selector4/1 -> Human Machine Interface (HMI)/9(HMI_Front_Camera_Blocked)  "<Carema_Status>"
  [LLOn_bsLLState] -> Bus Selector3/1
  Bus Selector5/1 -> Human Machine Interface (HMI)/1(HMI_stDACmode)  "<LKA_Mode>"
  Bus Selector1/1 -> Human Machine Interface (HMI)/5(HMI_R0_Quality)  "<R0_Q>"
  Bus Selector1/2 -> Human Machine Interface (HMI)/6(HMI_L0_Quality)  "<L0_Q>"
  Bus Selector2/1 -> Human Machine Interface (HMI)/7(HMI_EPSInfo)  "<bsEPSInfo>"
  [LLOn_bsLDWWarnInfo] -> Human Machine Interface (HMI)/4(HMI_LDWWarn)

== system G59_LKAS_Carsim/LLClb ==
  Bus Creator : BusCreator  Inputs=4
  ConstantClb : Subsystem
  LDWClb : Subsystem
  LKAClb : Subsystem
  LLSMConClb : Subsystem
  LLClb_bsLLClb : Outport
  wires:
  ConstantClb/1(ConstantClb) -> Bus Creator/4  "bsConstantClb"
  LLSMConClb/1(LLSMConClb) -> Bus Creator/1  "bsLLSMConClb"
  Bus Creator/1 -> LLClb_bsLLClb/1  "bsLLClb"
  LDWClb/1(LDWClb) -> Bus Creator/2  "bsLDWClb"
  LKAClb/1(LKAClb) -> Bus Creator/3  "bsLKAClb"

== system G59_LKAS_Carsim/LaneData ==
  LinePoints : Inport
  Bus Creator : BusCreator  Inputs=6
  Bus Creator1 : BusCreator  Inputs=6
  Cast To Single{1..20} (20 alike) : DataTypeConversion  OutDataTypeStr=single
  Constant : Constant  Value=3  OutDataTypeStr=single
  Constant1 : Constant  Value=3  OutDataTypeStr=single
  Demux : Demux
  Demux1 : Demux
  Demux2 : Demux  Outputs=20
  MATLAB Function : MATLAB Function  TreatAsAtomicUnit=on
  MATLAB Function1 : MATLAB Function  TreatAsAtomicUnit=on
  MATLAB Function2 : MATLAB Function  TreatAsAtomicUnit=on
  MinMax : MinMax  Function=max
  MinMax1 : MinMax  Function=max
  Mux{,1..3} (4 alike) : Mux  Inputs=5
  Unary Minus1 : UnaryMinus
  Unary Minus2 : UnaryMinus
  L0 : Outport
  R0 : Outport  Port=2
  wires:
  Constant/1 -> Bus Creator/6  "L0_Q"
  Cast To Single8/1 -> MATLAB Function/8(x8)
  Demux2/8 -> Cast To Single8/1
  Demux2/10 -> Cast To Single10/1
  Cast To Single2/1 -> MATLAB Function/2(x2)
  Demux2/6 -> Cast To Single6/1
  MATLAB Function/11(ly1) -> Mux2/1
  Demux2/11 -> Cast To Single11/1
  Demux2/4 -> Cast To Single4/1
  Cast To Single6/1 -> MATLAB Function/6(x6)
  Cast To Single7/1 -> MATLAB Function/7(x7)
  Demux1/2 -> Bus Creator1/2  "R0_C2"
  Demux2/19 -> Cast To Single19/1
  Demux/3 -> Bus Creator/3  "L0_C1"
  Cast To Single11/1 -> MATLAB Function/11(y1)
  Demux2/7 -> Cast To Single7/1
  MATLAB Function/18(ry3) -> Mux3/3
  Demux/4 -> Bus Creator/4  "L0_C0"
  Constant1/1 -> Bus Creator1/6  "R0_Q"
  Demux2/9 -> Cast To Single9/1
  Mux1/1 -> MATLAB Function2/1(x), MinMax1/1
  Mux3/1 -> Unary Minus1/1
  Demux2/1 -> Cast To Single1/1
  Demux1/4 -> Bus Creator1/4  "R0_C0"
  MATLAB Function/5(lx5) -> Mux/5
  Cast To Single19/1 -> MATLAB Function/19(y9)
  MATLAB Function1/1(p) -> Demux/1
  Mux/1 -> MinMax/1, MATLAB Function1/1(x)
  Cast To Single9/1 -> MATLAB Function/9(x9)
  Demux2/16 -> Cast To Single16/1
  Demux1/3 -> Bus Creator1/3  "R0_C1"
  MinMax/1 -> Bus Creator/5  "L0_VR"
  Cast To Single20/1 -> MATLAB Function/20(y10)
  Demux2/15 -> Cast To Single15/1
  MATLAB Function/10(rx5) -> Mux1/5
  MATLAB Function2/1(p) -> Demux1/1
  Demux2/3 -> Cast To Single3/1
  Cast To Single10/1 -> MATLAB Function/10(x10)
  Mux2/1 -> Unary Minus2/1
  MATLAB Function/7(rx2) -> Mux1/2
  MATLAB Function/14(ly4) -> Mux2/4
  MATLAB Function/3(lx3) -> Mux/3
  Demux2/13 -> Cast To Single13/1
  Demux2/14 -> Cast To Single14/1
  MATLAB Function/17(ry2) -> Mux3/2
  MATLAB Function/4(lx4) -> Mux/4
  Demux2/2 -> Cast To Single2/1
  Demux2/18 -> Cast To Single18/1
  Cast To Single15/1 -> MATLAB Function/15(y5)
  Demux2/12 -> Cast To Single12/1
  MATLAB Function/9(rx4) -> Mux1/4
  MATLAB Function/6(rx1) -> Mux1/1
  Demux2/17 -> Cast To Single17/1
  Demux1/1 -> Bus Creator1/1  "R0_C3"
  MATLAB Function/12(ly2) -> Mux2/2
  MATLAB Function/16(ry1) -> Mux3/1
  MATLAB Function/15(ly5) -> Mux2/5
  Demux2/5 -> Cast To Single5/1
  Demux/1 -> Bus Creator/1  "L0_C3"
  Cast To Single4/1 -> MATLAB Function/4(x4)
  MATLAB Function/1(lx1) -> Mux/1
  Cast To Single17/1 -> MATLAB Function/17(y7)
  Demux/2 -> Bus Creator/2  "L0_C2"
  MATLAB Function/19(ry4) -> Mux3/4
  MATLAB Function/2(lx2) -> Mux/2
  MinMax1/1 -> Bus Creator1/5  "R0_VR"
  Cast To Single16/1 -> MATLAB Function/16(y6)
  Cast To Single1/1 -> MATLAB Function/1(x1)
  Cast To Single14/1 -> MATLAB Function/14(y4)
  MATLAB Function/8(rx3) -> Mux1/3
  Unary Minus1/1 -> MATLAB Function2/2(y)  "R0_C0"
  Cast To Single12/1 -> MATLAB Function/12(y2)
  Unary Minus2/1 -> MATLAB Function1/2(y)  "L0_C0"
  MATLAB Function/20(ry5) -> Mux3/5
  Cast To Single13/1 -> MATLAB Function/13(y3)
  Cast To Single5/1 -> MATLAB Function/5(x5)
  Cast To Single18/1 -> MATLAB Function/18(y8)
  Demux2/20 -> Cast To Single20/1
  Bus Creator/1 -> L0/1
  MATLAB Function/13(ly3) -> Mux2/3
  Cast To Single3/1 -> MATLAB Function/3(x3)
  LinePoints/1 -> Demux2/1
  Bus Creator1/1 -> R0/1

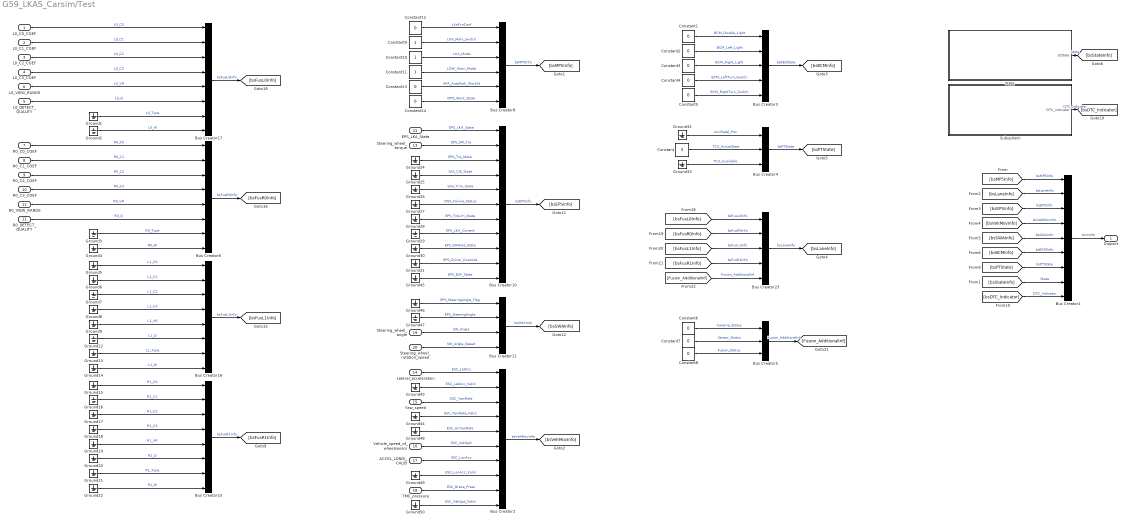
== system G59_LKAS_Carsim/Test ==
  L0_C0_COEF : Inport
  L0_C1_COEF : Inport  Port=2
  L0_C2_COEF : Inport  Port=3
  L0_C3_COEF : Inport  Port=4
  L0_DETECT_QUALITY : Inport  Port=5
  L0_VIEW_RANGE : Inport  Port=6
  R0_C0_COEF : Inport  Port=7
  R0_C1_COEF : Inport  Port=8
  R0_C2_COEF : Inport  Port=9
  R0_C3_COEF : Inport  Port=10
  R0_DETECT_QUALITY : Inport  Port=11
  R0_VIEW_RANGE : Inport  Port=12
  Steering_wheel_torque : Inport  Port=13
  Lateral_acceleration : Inport  Port=14
  Yaw_speed : Inport  Port=15
  Vehicle_speed_of_wheelsensor : Inport  Port=16
  ACCEL_LONGI_CALIB : Inport  Port=17
  TMC_pressure : Inport  Port=18
  Steering_wheel_angle : Inport  Port=19
  Steering_wheel_rotation_speed : Inport  Port=20
  EPS_LKA_State : Inport  Port=21
  Bus Creator1 : BusCreator  Inputs=9
  Bus Creator10 : BusCreator  Inputs=11
  Bus Creator11 : BusCreator  Inputs=4
  Bus Creator{6,15..17} (4 alike) : BusCreator  Inputs=8
  Bus Creator2 : BusCreator  Inputs=10
  Bus Creator23 : BusCreator  Inputs=5
  Bus Creator3 : BusCreator  Inputs=5
  Bus Creator4 : BusCreator  Inputs=3
  Bus Creator5 : BusCreator  Inputs=3
  Bus Creator8 : BusCreator  Inputs=6
  Constant : Constant  Value=3  OutDataTypeStr=uint8
  Constant{1..8,12..14} (11 alike) : Constant  Value=0  OutDataTypeStr=uint8
  Constant10 : Constant  OutDataTypeStr=uint8
  Constant11 : Constant  OutDataTypeStr=uint8
  Constant9 : Constant  OutDataTypeStr=uint8
  Ground{1..9,12..22,24..33,43..50} (38 alike) : Ground
  State : Subsystem
  Subsystem : Subsystem
  Outport : Outport
  wires:
  Steering_wheel_angle/1 -> Bus Creator11/3  "SW_Angle"
  State/1(stState) -> [bsStateInfo]  "State"
  R0_DETECT_QUALITY/1 -> Bus Creator6/6  "R0_Q"
  R0_C2_COEF/1 -> Bus Creator6/3  "R0_C2"
  R0_C1_COEF/1 -> Bus Creator6/2  "R0_C1"
  L0_C0_COEF/1 -> Bus Creator17/1  "L0_C0"
  L0_C2_COEF/1 -> Bus Creator17/3  "L0_C2"
  L0_C3_COEF/1 -> Bus Creator17/4  "L0_C3"
  R0_C0_COEF/1 -> Bus Creator6/1  "R0_C0"
  Subsystem/1(DTC_Indicator) -> [bsDTC_Indicator]  "DTC_Indicator"
  Ground9/1 -> Bus Creator16/5  "L1_VR"
  Ground22/1 -> Bus Creator15/8  "R1_W"
  Bus Creator6/1 -> [bsFusR0Info]  "bsFusR0Info"
  Ground4/1 -> Bus Creator6/8  "R0_W"
  Bus Creator15/1 -> [bsFusR1Info]  "bsFusR1Info"
  R0_C3_COEF/1 -> Bus Creator6/4  "R0_C3"
  Ground1/1 -> Bus Creator17/7  "L0_Type"
  Ground18/1 -> Bus Creator15/4  "R1_C3"
  Ground15/1 -> Bus Creator15/1  "R1_C0"
  Bus Creator17/1 -> [bsFusL0Info]  "bsFusL0Info"
  Ground12/1 -> Bus Creator16/6  "L1_Q"
  Ground2/1 -> Bus Creator17/8  "L0_W"
  Ground19/1 -> Bus Creator15/5  "R1_VR"
  Ground16/1 -> Bus Creator15/2  "R1_C1"
  Ground20/1 -> Bus Creator15/6  "R1_Q"
  Ground5/1 -> Bus Creator16/1  "L1_C0"
  Ground6/1 -> Bus Creator16/2  "L1_C1"
  Ground14/1 -> Bus Creator16/8  "L1_W"
  Ground8/1 -> Bus Creator16/4  "L1_C3"
  Ground7/1 -> Bus Creator16/3  "L1_C2"
  Ground3/1 -> Bus Creator6/7  "R0_Type"
  L0_DETECT_QUALITY/1 -> Bus Creator17/6  "L0_Q"
  R0_VIEW_RANGE/1 -> Bus Creator6/5  "R0_VR"
  L0_VIEW_RANGE/1 -> Bus Creator17/5  "L0_VR"
  Ground21/1 -> Bus Creator15/7  "R1_Type"
  L0_C1_COEF/1 -> Bus Creator17/2  "L0_C1"
  Bus Creator16/1 -> [bsFusL1Info]  "bsFusL1Info"
  Ground13/1 -> Bus Creator16/7  "L1_Type"
  Ground17/1 -> Bus Creator15/3  "R1_C2"
  Constant10/1 -> Bus Creator8/3  "LKA_Mode"
  Constant11/1 -> Bus Creator8/4  "LDW_Warn_Mode"
  Constant13/1 -> Bus Creator8/5  "APA_AutoPark_WorkSt"
  Constant12/1 -> Bus Creator8/1  "LkaFcnConf"
  Constant9/1 -> Bus Creator8/2  "LKA_Main_Switch"
  Constant14/1 -> Bus Creator8/6  "MP5_Work_State"
  Bus Creator8/1 -> [bsMP5Info]  "bsMP5Info"
  Bus Creator10/1 -> [bsEPSInfo]  "bsEPSInfo"
  Ground26/1 -> Bus Creator10/5  "SAS_Trim_State"
  Ground45/1 -> Bus Creator10/11  "EPS_ESA_State"
  EPS_LKA_State/1 -> Bus Creator10/1  "EPS_LKA_State"
  Ground30/1 -> Bus Creator10/9  "EPS_SWHold_State"
  Ground31/1 -> Bus Creator10/10  "EPS_Driver_Override"
  Ground28/1 -> Bus Creator10/7  "EPS_TrqLim_State"
  Ground24/1 -> Bus Creator10/3  "EPS_Trq_State"
  Steering_wheel_torque/1 -> Bus Creator10/2  "EPS_SW_Trq"
  Ground29/1 -> Bus Creator10/8  "EPS_LKA_Current"
  Ground27/1 -> Bus Creator10/6  "SWS_Failure_Status"
  Ground25/1 -> Bus Creator10/4  "SAS_Clb_State"
  Steering_wheel_rotation_speed/1 -> Bus Creator11/4  "SW_Angle_Speed"
  Ground47/1 -> Bus Creator11/2  "EPS_SteeringAngle"
  Ground46/1 -> Bus Creator11/1  "EPS_SteeringAngle_Flag"
  Bus Creator11/1 -> [bsSWAInfo]  "bsSWAInfo"
  Yaw_speed/1 -> Bus Creator2/3  "ESC_YawRate"
  Ground44/1 -> Bus Creator2/4  "ESC_YawRate_Valid"
  Ground48/1 -> Bus Creator2/5  "ESC_UnYawRate"
  TMC_pressure/1 -> Bus Creator2/9  "ESC_Brake_Press"
  ACCEL_LONGI_CALIB/1 -> Bus Creator2/7  "ESC_LonAcc"
  Vehicle_speed_of_wheelsensor/1 -> Bus Creator2/6  "ESC_VehSpd"
  Lateral_acceleration/1 -> Bus Creator2/1  "ESC_LatAcc"
  Ground50/1 -> Bus Creator2/10  "ESC_VehSpd_Valid"
  Ground43/1 -> Bus Creator2/2  "ESC_LatAcc_Valid"
  Bus Creator2/1 -> [bsVehMovInfo]  "bsVehMovInfo"
  Ground49/1 -> Bus Creator2/8  "ESC_LonAcc_Valid"
  Constant3/1 -> Bus Creator3/3  "BCM_Right_Light"
  Constant4/1 -> Bus Creator3/4  "BCM_LeftTurn_Switch"
  Bus Creator3/1 -> [bsBCMInfo]  "bsBESState"
  Constant1/1 -> Bus Creator3/1  "BCM_Double_Light"
  Constant2/1 -> Bus Creator3/2  "BCM_Left_Light"
  Constant5/1 -> Bus Creator3/5  "BCM_RightTurn_Switch"
  Ground33/1 -> Bus Creator4/3  "TCU_Available"
  Constant/1 -> Bus Creator4/2  "TCU_ActualGear"
  Bus Creator4/1 -> [bsPTState]  "bsPTState"
  Ground32/1 -> Bus Creator4/1  "AccPedal_Pos"
  [Fusion_AdditionalInf] -> Bus Creator23/5  "Fusion_AdditionalInf"
  Bus Creator23/1 -> [bsLaneInfo]  "bsLaneInfo"
  [bsFusL1Info] -> Bus Creator23/3  "bsFusL1Info"
  [bsFusR0Info] -> Bus Creator23/2  "bsFusR0Info"
  [bsFusL0Info] -> Bus Creator23/1  "bsFusL0Info"
  [bsFusR1Info] -> Bus Creator23/4  "bsFusR1Info"
  Constant6/1 -> Bus Creator5/1  "Carema_Status"
  Constant8/1 -> Bus Creator5/3  "Fusion_Status"
  Constant7/1 -> Bus Creator5/2  "Sensor_Status"
  Bus Creator5/1 -> [Fusion_AdditionalInf]  "Fusion_AdditionalInf"
  [bsVehMovInfo] -> Bus Creator1/4  "bsVehMovInfo"
  [bsMP5Info] -> Bus Creator1/1  "bsMP5Info"
  [bsDTC_Indicator] -> Bus Creator1/9  "DTC_Indicator"
  [bsLaneInfo] -> Bus Creator1/2  "bsLaneInfo"
  [bsBCMInfo] -> Bus Creator1/6  "bsBCMInfo"
  [bsPTState] -> Bus Creator1/7  "bsPTState"
  [bsEPSInfo] -> Bus Creator1/3  "bsEPSInfo"
  [bsStateInfo] -> Bus Creator1/8  "State"
  [bsSWAInfo] -> Bus Creator1/5  "bsSWAInfo"
  Bus Creator1/1 -> Outport/1  "bsInInfo"

== system G59_LKAS_Carsim/LL/Fault_Diagnostic ==
  bsInInfo : Inport
  Bus Creator : BusCreator  Inputs=2
  Bus Creator1 : BusCreator  Inputs=10
  Bus Selector3 : BusSelector  OutputSignals=DTC_Indicator.LKAS_BSWDTC_Status
  Bus Selector4 : BusSelector  OutputSignals=bsVehMovInfo.ESC_VehSpd_Valid,bsEPSInfo.EPS_LKA_State,bsEPSInfo.SAS_Clb_State,bsEPSInfo.SAS_Trim_State,bsPTState.TCU_ActualGear,bsEPSInfo.EPS_TrqLim_State,bsEPSInfo.EPS_Trq_State,bsVehMovInfo.ESC_LatAcc_Valid,bsVehMovInfo.ESC_YawRate_Valid,bsVehMovInfo.ESC_LonAcc_Valid
  Compare To Constant26 : simulink/Logic and Bit Operations/Compare To Constant  relop=~=  const=1  OutDataTypeStr=boolean
  Compare To Constant27 : simulink/Logic and Bit Operations/Compare To Constant  relop===  const=4  OutDataTypeStr=boolean
  Compare To Constant29 : simulink/Logic and Bit Operations/Compare To Constant  relop===  const=0  OutDataTypeStr=boolean
  Compare To Constant{30,36..39} (5 alike) : simulink/Logic and Bit Operations/Compare To Constant  relop===  const=1  OutDataTypeStr=boolean
  Compare To Constant34 : simulink/Logic and Bit Operations/Compare To Constant  relop=>  const=3  OutDataTypeStr=boolean
  Compare To Constant35 : simulink/Logic and Bit Operations/Compare To Constant  relop===  const=0  OutDataTypeStr=boolean
  bsSignalFault : Outport
  wires:
  Compare To Constant27/1 -> Bus Creator1/2  "Event_FaulEPSLKASt"
  Bus Creator1/1 -> Bus Creator/2  "LKAS_ASWDTC_Status"
  Compare To Constant39/1 -> Bus Creator1/10  "Event_FaulLonAcc"
  Compare To Constant38/1 -> Bus Creator1/9  "Event_FaulYawRate"
  Compare To Constant37/1 -> Bus Creator1/8  "Event_FaulLatAcc"
  Compare To Constant36/1 -> Bus Creator1/7  "Event_FaulEPSTrqSt"
  Compare To Constant34/1 -> Bus Creator1/5  "Event_FaulTCUGear"
  Compare To Constant35/1 -> Bus Creator1/6  "Event_FaulTrqLim"
  Compare To Constant30/1 -> Bus Creator1/4  "Event_FaulSASTrim"
  Bus Selector4/10 -> Compare To Constant39/1  "<ESC_LonAcc_Valid>"
  Bus Selector4/9 -> Compare To Constant38/1  "<ESC_YawRate_Valid>"
  Bus Selector4/8 -> Compare To Constant37/1  "<ESC_LatAcc_Valid>"
  Bus Selector4/7 -> Compare To Constant36/1  "<EPS_Trq_State>"
  Bus Selector4/6 -> Compare To Constant35/1  "<EPS_TrqLim_State>"
  Bus Selector4/5 -> Compare To Constant34/1  "<TCU_ActualGear>"
  Bus Selector4/4 -> Compare To Constant30/1  "<SAS_Trim_State>"
  Compare To Constant29/1 -> Bus Creator1/3  "Event_FaulSASClb"
  Bus Selector4/3 -> Compare To Constant29/1  "<SAS_Clb_State>"
  Bus Selector4/2 -> Compare To Constant27/1  "<EPS_LKA_State>"
  Compare To Constant26/1 -> Bus Creator1/1  "Event_FaulVehSpeed"
  Bus Selector4/1 -> Compare To Constant26/1  "<ESC_VehSpd_Valid>"
  bsInInfo/1 -> Bus Selector3/1, Bus Selector4/1
  Bus Selector3/1 -> Bus Creator/1  "<LKAS_BSWDTC_Status>"
  Bus Creator/1 -> bsSignalFault/1

== system G59_LKAS_Carsim/LL/Human Machine Interface (HMI) ==
  HMI_stDACmode : Inport
  HMI_LKA_STATE : Inport  Port=2
  HMI_LDW_STATE : Inport  Port=3
  HMI_LDWWarn : Inport  Port=4
  HMI_R0_Quality : Inport  Port=5
  HMI_L0_Quality : Inport  Port=6
  HMI_EPSInfo : Inport  Port=7
  HMI_camera_common_fault : Inport  Port=8
  HMI_Front_Camera_Blocked : Inport  Port=9
  HMI_stFaultCSyn : Inport  Port=10
  Bus Creator2 : BusCreator  Inputs=7
  Cast To Single{,1..6} (7 alike) : DataTypeConversion  OutDataTypeStr=uint8
  HMI_Popup_Status : MATLAB Function  TreatAsAtomicUnit=on
  Hands_Off_Warning : MATLAB Function  TreatAsAtomicUnit=on
  LDW_Flag : MATLAB Function  TreatAsAtomicUnit=on
  LDW_Status_Display : MATLAB Function  TreatAsAtomicUnit=on
  LKA_Status_Display : MATLAB Function  TreatAsAtomicUnit=on
  LKA_action_indication : MATLAB Function  TreatAsAtomicUnit=on
  Subsystem : Subsystem
  Vehicle_Lane_Display : MATLAB Function  TreatAsAtomicUnit=on
  HMI_LDWLKA : Outport
  wires:
  HMI_LDWWarn/1 -> LDW_Flag/3(HMI_LDWWarnInfo)
  Subsystem/2(HandsOff15s) -> Hands_Off_Warning/1(HandsOff)
  Subsystem/1(HandsOff10s) -> HMI_Popup_Status/3(HandsOff)
  HMI_EPSInfo/1 -> Subsystem/3(EPSInfo)  "HMI_EPSInfo"
  HMI_camera_common_fault/1 -> HMI_Popup_Status/4(camera_common_fault)  "HMI_camera_common_fault"
  HMI_R0_Quality/1 -> Vehicle_Lane_Display/4(R0_Quality)  "HMI_R0_Quality"
  HMI_Front_Camera_Blocked/1 -> HMI_Popup_Status/5(Front_Camera_Blocked)  "HMI_Front_Camera_Blocked"
  HMI_stDACmode/1 -> LKA_Status_Display/1(stDACmode), LDW_Flag/1(HMI_stDACmode), HMI_Popup_Status/1(stDACmode), LKA_action_indication/1(stDACmode), LDW_Status_Display/1(stDACmode), Vehicle_Lane_Display/1(stDACmode)  "HMI_stDACmode"
  HMI_L0_Quality/1 -> Vehicle_Lane_Display/5(L0_Quality)  "HMI_L0_Quality"
  HMI_stFaultCSyn/1 -> HMI_Popup_Status/6(stFaultCSyn)  "HMI_stFaultCSyn"
  HMI_LDW_STATE/1 -> LDW_Status_Display/2(LDW_STATE), Vehicle_Lane_Display/3(LDW_STATE), Subsystem/1(LDW_STATE)  "HMI_LDW_STATE"
  HMI_LKA_STATE/1 -> LKA_Status_Display/2(LKA_STATE), LDW_Flag/2(HMI_LKA_STATE), HMI_Popup_Status/2(LKA_STATE), LKA_action_indication/2(LKA_STATE), Vehicle_Lane_Display/2(LKA_STATE), Subsystem/2(LKA_STATE)  "HMI_LKA_STATE"
  Cast To Single4/1 -> Bus Creator2/5  "Hands_Off_Warning"
  LKA_action_indication/1(LKA_Action_Indication) -> Cast To Single5/1  "LKA_Action_Indication"
  Cast To Single6/1 -> Bus Creator2/7  "HMI_Popup_Status"
  Cast To Single/1 -> Bus Creator2/1  "Vehicle_Lane_Display"
  Vehicle_Lane_Display/1(Vehicle_Lane_Display) -> Cast To Single/1  "Vehicle_Lane_Display"
  Cast To Single3/1 -> Bus Creator2/4  "LDW_Flag"
  LKA_Status_Display/1(LKA_Status_Display) -> Cast To Single2/1  "LKA_Status_Display"
  Cast To Single1/1 -> Bus Creator2/2  "LDW_Status_Display"
  HMI_Popup_Status/1(HMI_Popup_Status) -> Cast To Single6/1  "HMI_Popup_Status"
  LDW_Status_Display/1(LDW_Status_Display) -> Cast To Single1/1  "LDW_Status_Display"
  LDW_Flag/1(LDW_Flag) -> Cast To Single3/1  "LDW_Flag"
  Cast To Single2/1 -> Bus Creator2/3  "LKA_Status_Display"
  Cast To Single5/1 -> Bus Creator2/6  "LKA_Action_Indication"
  Hands_Off_Warning/1(Hands_Off_Warning) -> Cast To Single4/1  "Hands_Off_Warning"
  Bus Creator2/1 -> HMI_LDWLKA/1

== system G59_LKAS_Carsim/LL/LL Inputs Mapping ==
  bsInInfo : Inport
  Bus Creator : BusCreator  Inputs=7
  Bus Selector : BusSelector  OutputSignals=bsMP5Info,bsLaneInfo,bsEPSInfo,bsVehMovInfo,bsSWAInfo,bsBCMInfo,bsPTState
  bsBCMInfo : Subsystem
  bsEPSInfo : Subsystem
  bsLaneInfo : Subsystem
  bsMP5Info : Subsystem
  bsPTState : Subsystem
  bsSWAInfo : Subsystem
  bsVehMovInfo : Subsystem
  bsInfo : Outport
  wires:
  bsInInfo/1 -> Bus Selector/1
  Bus Creator/1 -> bsInfo/1
  Bus Selector/2 -> bsLaneInfo/1(bsLaneInfoIn)  "<bsLaneInfo>"
  Bus Selector/3 -> bsEPSInfo/1(bsEPSInfoIn)  "<bsEPSInfo>"
  bsEPSInfo/1(bsEPSInfoOut) -> Bus Creator/3  "bsEPSInfo"
  Bus Selector/4 -> bsVehMovInfo/1(bsVehMovInfoIn)  "<bsVehMovInfo>"
  bsVehMovInfo/1(bsVehMovInfoOut) -> Bus Creator/4  "bsVehMovInfo"
  Bus Selector/5 -> bsSWAInfo/1(bsSWAInfoIn)  "<bsSWAInfo>"
  Bus Selector/6 -> bsBCMInfo/1(bsBCMInfoIn)  "<bsBCMInfo>"
  Bus Selector/1 -> bsMP5Info/1(bsMP5InfoIn)  "<bsMP5Info>"
  bsMP5Info/1(bsMP5InfoOut) -> Bus Creator/1  "bsMP5Info"
  bsBCMInfo/1(bsBCMInfoOut) -> Bus Creator/6  "bsBCMInfo"
  Bus Selector/7 -> bsPTState/1(bsPTStateIn)  "<bsPTState>"
  bsPTState/1(bsPTStateOut) -> Bus Creator/7  "bsPTState"
  bsLaneInfo/1(bsLaneInfoOut) -> Bus Creator/2  "bsLaneInfo"
  bsSWAInfo/1(bsSWAInfoOut) -> Bus Creator/5  "bsSWAInfo"

== system G59_LKAS_Carsim/LL/LLOn ==
  bsInInfo : Inport
  bsLLClb : Inport  Port=2
  bsSignalFault : Inport  Port=3
  Enable : EnablePort  StatesWhenEnabling=reset
      settings: AttributesFormatString=states = %<StatesWhenEnabling>
  LDW : Subsystem  Description=|  TreatAsAtomicUnit=on
      | Block Name: Lane Departure Warning
      | Ab.: LDW
      | No.: 1.3.0.0
      | Rev: 0.0.1
      | Update Date: 19-3-26
  LKA : Subsystem  Description=|  TreatAsAtomicUnit=on
      | Block Name: Lane Keeping Assistance
      | Ab.: LKA
      | No.: 1.2.0.0
      | Rev: 0.0.1
      | Update Date: 19-5-13
  LKA Input Processing (LKAInP) : Subsystem
  LL State Determination (LLStateDet) : Subsystem
  LL_Mon : Subsystem
  bsLLState : Outport  OutputWhenDisabled=reset  InitialOutput=0
      settings: AttributesFormatString=%<OutputWhenDisabled> = %<InitialOutput>
  LDW_Flag : Outport  Port=2  OutputWhenDisabled=reset  InitialOutput=0
      settings: AttributesFormatString=%<OutputWhenDisabled> = %<InitialOutput>
  phiSWACmd : Outport  Port=3  OutputWhenDisabled=reset  InitialOutput=0
      settings: AttributesFormatString=%<OutputWhenDisabled> = %<InitialOutput>
  M : Outport  Port=4  OutputWhenDisabled=reset  InitialOutput=0
      settings: AttributesFormatString=%<OutputWhenDisabled> = %<InitialOutput>
  LLMon : Outport  Port=5
      settings: AttributesFormatString=%<OutputWhenDisabled> = %<InitialOutput>
  wires:
  LL State Determination (LLStateDet)/4(Disable_Reason) -> LL_Mon/1(Disable_Reason)
  [ActFlg] -> LKA Input Processing (LKAInP)/3(In3)
  [bsLLClb] -> LKA/3(LKA_bsLKAClb)
  LL_Mon/1(LLMon) -> LLMon/1
  [LKAMon] -> LL_Mon/2(LKAMon)
  LKA/4(LKAMon) -> [LKAMon]
  LKA/3(LKA_M) -> M/1  "OutputM"
  bsSignalFault/1 -> LL State Determination (LLStateDet)/5(LLStateDet_SignalFault)
  LKA/1(LKA_ExitFlg) -> [ExitFlg]
  LKA/2(LKA_phiSWACmd) -> phiSWACmd/1  "OutputSWACmd"
  [ExitFlg] -> LL State Determination (LLStateDet)/4(LLStateDet_stExitFlg)
  bsInInfo/1 -> LKA Input Processing (LKAInP)/1(LKAInP_bsInInfoSyn), LL State Determination (LLStateDet)/1(LLStateDet_bsInInfoSyn), LDW/1(LDW_bsInInfoSyn), LKA/1(LKA_bsInInfoSyn)
  LDW/1(LDW_Flag) -> LDW_Flag/1  "LDW_Flag"
  LL State Determination (LLStateDet)/3(LLStateDet_stLKAActvFlg) -> [ActFlg], LKA/Enable
  bsLLClb/1 -> [bsLLClb]
  LKA Input Processing (LKAInP)/1(LKAInP_bsLKAInPInfo) -> LKA/2(LKA_bsLKAInPInfo), LL State Determination (LLStateDet)/2(LLStateDet_bsLKAInPInfo)
  [bsLLClb] -> LDW/2(LDW_bsLDWClb)
  LL State Determination (LLStateDet)/1(LLStateDet_bsLLState) -> bsLLState/1
  [bsLLClb] -> LKA Input Processing (LKAInP)/2(LKAInP_bsLLClb)
  [bsLLClb] -> LL State Determination (LLStateDet)/3(LLStateDet_bsLLClb)
  LL State Determination (LLStateDet)/2(LLStateDet_stLDWActvFlg) -> LDW/Enable

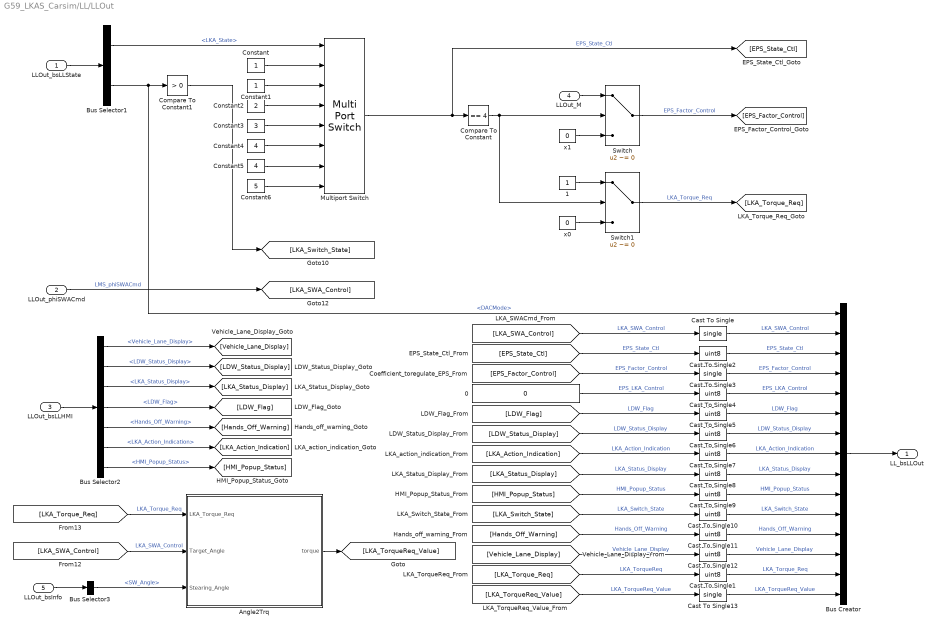
== system G59_LKAS_Carsim/LL/LLOut ==
  LLOut_bsLLState : Inport
  LLOut_phiSWACmd : Inport  Port=2
  LLOut_bsLLHMI : Inport  Port=3
  LLOut_M : Inport  Port=4
  LLOut_bsInfo : Inport  Port=5
  0 : Constant  Value=0  OutDataTypeStr=uint16
      settings: AttributesFormatString=DT: %<OutDataTypeStr>
  1 : Constant  OutDataTypeStr=uint8
      settings: AttributesFormatString=DT: %<OutDataTypeStr>
  Angle2Trq : Subsystem
  Bus Creator : BusCreator  Inputs=15
  Bus Selector1 : BusSelector  OutputSignals=LKA_State,DACMode
  Bus Selector2 : BusSelector  OutputSignals=Vehicle_Lane_Display,LDW_Status_Display,LKA_Status_Display,LDW_Flag,Hands_Off_Warning,LKA_Action_Indication,HMI_Popup_Status
  Bus Selector3 : BusSelector  OutputSignals=bsSWAInfo.SW_Angle
  Cast To Single : DataTypeConversion  OutDataTypeStr=single
  Cast To Single{1..2,4..12} (11 alike) : DataTypeConversion  OutDataTypeStr=uint8
  Cast To Single13 : DataTypeConversion  OutDataTypeStr=single
  Cast To Single3 : DataTypeConversion  OutDataTypeStr=single
  Compare To Constant : simulink/Logic and Bit Operations/Compare To Constant  relop===  const=4  OutDataTypeStr=boolean
  Compare To Constant1 : simulink/Logic and Bit Operations/Compare To Constant  relop=>  const=0  OutDataTypeStr=boolean
  Constant : Constant  OutDataTypeStr=uint8
  Constant1 : Constant  OutDataTypeStr=uint8
  Constant2 : Constant  Value=2  OutDataTypeStr=uint8
  Constant3 : Constant  Value=3  OutDataTypeStr=uint8
  Constant4 : Constant  Value=4  OutDataTypeStr=uint8
  Constant5 : Constant  Value=4  OutDataTypeStr=uint8
  Constant6 : Constant  Value=5  OutDataTypeStr=uint8
  Multiport Switch : MultiPortSwitch  DataPortOrder=Zero-based contiguous  Inputs=7  zeroidx=on
  Switch : Switch  Criteria=u2 ~= 0
      settings: AttributesFormatString=%<Criteria>
  Switch1 : Switch  Criteria=u2 ~= 0
      settings: AttributesFormatString=%<Criteria>
  x0 : Constant  Value=0  OutDataTypeStr=uint8
      settings: AttributesFormatString=DT: %<OutDataTypeStr>
  x1 : Constant  Value=0  OutDataTypeStr=uint8
      settings: AttributesFormatString=DT: %<OutDataTypeStr>
  LL_bsLLOut : Outport
      settings: AttributesFormatString=Disable Action: %<OutputWhenDisabled>
  wires:
  x1/1 -> Switch/3
  Bus Selector3/1 -> Angle2Trq/3(Stearing_Angle)  "<SW_Angle>"
  LLOut_bsInfo/1 -> Bus Selector3/1
  Angle2Trq/1(torque) -> [LKA_TorqueReq_Value]
  [LKA_SWA_Control] -> Angle2Trq/2(Target_Angle)  "LKA_SWA_Control"
  [LKA_Torque_Req] -> Angle2Trq/1(LKA_Torque_Req)  "LKA_Torque_Req"
  LLOut_phiSWACmd/1 -> [LKA_SWA_Control]  "LMS_phiSWACmd"
  x0/1 -> Switch1/3
  1/1 -> Switch1/1
  Switch1/1 -> [LKA_Torque_Req]  "LKA_Torque_Req"
  Bus Selector2/1 -> [Vehicle_Lane_Display]  "<Vehicle_Lane_Display>"
  Bus Selector2/7 -> [HMI_Popup_Status]  "<HMI_Popup_Status>"
  Bus Selector2/3 -> [LKA_Status_Display]  "<LKA_Status_Display>"
  Bus Selector2/4 -> [LDW_Flag]  "<LDW_Flag>"
  LLOut_bsLLHMI/1 -> Bus Selector2/1
  Bus Selector2/2 -> [LDW_Status_Display]  "<LDW_Status_Display>"
  Bus Selector2/6 -> [LKA_Action_Indication]  "<LKA_Action_Indication>"
  Bus Selector2/5 -> [Hands_Off_Warning]  "<Hands_Off_Warning>"
  Constant/1 -> Multiport Switch/2
  Constant5/1 -> Multiport Switch/7
  Cast To Single11/1 -> Bus Creator/12  "Hands_Off_Warning"
  LLOut_M/1 -> Switch/1
  Cast To Single9/1 -> Bus Creator/10  "HMI_Popup_Status"
  Constant4/1 -> Multiport Switch/6
  Compare To Constant1/1 -> [LKA_Switch_State]
  LLOut_bsLLState/1 -> Bus Selector1/1
  Constant1/1 -> Multiport Switch/3
  [EPS_State_Ctl] -> Cast To Single2/1  "EPS_State_Ctl"
  Cast To Single12/1 -> Bus Creator/13  "Vehicle_Lane_Display"
  Cast To Single6/1 -> Bus Creator/7  "LDW_Status_Display"
  Switch/1 -> [EPS_Factor_Control]  "EPS_Factor_Control"
  Multiport Switch/1 -> Compare To Constant/1, [EPS_State_Ctl]  "EPS_State_Ctl"
  Constant3/1 -> Multiport Switch/5
  Cast To Single3/1 -> Bus Creator/4  "EPS_Factor_Control"
  Bus Creator/1 -> LL_bsLLOut/1
  Cast To Single2/1 -> Bus Creator/3  "EPS_State_Ctl"
  Constant2/1 -> Multiport Switch/4
  Bus Selector1/2 -> Compare To Constant1/1, Bus Creator/1  "<DACMode>"
  Cast To Single10/1 -> Bus Creator/11  "LKA_Switch_State"
  Cast To Single4/1 -> Bus Creator/5  "EPS_LKA_Control"
  Cast To Single8/1 -> Bus Creator/9  "LKA_Status_Display"
  [Hands_Off_Warning] -> Cast To Single11/1  "Hands_Off_Warning"
  [LKA_Switch_State] -> Cast To Single10/1  "LKA_Switch_State"
  [LDW_Status_Display] -> Cast To Single6/1  "LDW_Status_Display"
  Cast To Single/1 -> Bus Creator/2  "LKA_SWA_Control"
  [LKA_SWA_Control] -> Cast To Single/1  "LKA_SWA_Control"
  [LKA_Status_Display] -> Cast To Single8/1  "LKA_Status_Display"
  Bus Selector1/1 -> Multiport Switch/1  "<LKA_State>"
  [HMI_Popup_Status] -> Cast To Single9/1  "HMI_Popup_Status"
  Cast To Single5/1 -> Bus Creator/6  "LDW_Flag"
  Constant6/1 -> Multiport Switch/8
  [LKA_Action_Indication] -> Cast To Single7/1  "LKA_Action_Indication"
  [EPS_Factor_Control] -> Cast To Single3/1  "EPS_Factor_Control"
  [LDW_Flag] -> Cast To Single5/1  "LDW_Flag"
  0/1 -> Cast To Single4/1  "EPS_LKA_Control"
  [Vehicle_Lane_Display] -> Cast To Single12/1  "Vehicle_Lane_Display"
  Compare To Constant/1 -> Switch1/2, Switch/2
  Cast To Single7/1 -> Bus Creator/8  "LKA_Action_Indication"
  [LKA_Torque_Req] -> Cast To Single1/1  "LKA_TorqueReq"
  Cast To Single1/1 -> Bus Creator/14  "LKA_Torque_Req"
  [LKA_TorqueReq_Value] -> Cast To Single13/1  "LKA_TorqueReq_Value"
  Cast To Single13/1 -> Bus Creator/15  "LKA_TorqueReq_Value"

== system G59_LKAS_Carsim/LLClb/ConstantClb ==
  Bus Creator : BusCreator  Inputs=6
  Data Type Conversion{2..4,6,13,22} (6 alike) : DataTypeConversion  OutDataTypeStr=single
  LKA_CarWidth=1.8 : Constant  Value=LKA_CarWidth
  LKA_SampleTime=0.01 : Constant  Value=LKA_SampleTime  OutDataTypeStr=single
  LKA_StrRatio_C=15.3 : Constant  Value=LKA_StrRatio_C
  LKA_Veh2CamL_C=1.56 : Constant  Value=LKA_Veh2CamL_C
  LKA_Veh2CamW_C=0.9 : Constant  Value=LKA_Veh2CamW_C  OutDataTypeStr=single
  LKA_WhlBaseL_C=2.65 : Constant  Value=LKA_WhlBaseL_C
  Switch{,1..3,11,19} (6 alike) : Switch  Criteria=u2 ~= 0  OutDataTypeStr=single
  ConstantClb : Outport
  wires:
  LKA_SampleTime=0.01/1 -> Switch19/3  "LKA_SampleTime"
  Data Type Conversion3/1 -> Switch19/1, Switch19/2
  Switch19/1 -> Bus Creator/1  "LKA_SampleTime"
  Switch2/1 -> Bus Creator/4  "LKA_WhlBaseL_C"
  Switch/1 -> Bus Creator/2  "LKA_Veh2CamW_C"
  Switch1/1 -> Bus Creator/3  "LKA_Veh2CamL_C"
  Switch11/1 -> Bus Creator/6  "LKA_CarWidth"
  Switch3/1 -> Bus Creator/5  "LKA_StrRatio_C"
  Bus Creator/1 -> ConstantClb/1
  LKA_CarWidth=1.8/1 -> Switch11/3  "LKA_CarWidth"
  Data Type Conversion22/1 -> Switch11/2, Switch11/1
  LKA_StrRatio_C=15.3/1 -> Switch3/3  "LKA_StrRatio_C"
  Data Type Conversion6/1 -> Switch3/2, Switch3/1
  Data Type Conversion4/1 -> Switch2/2, Switch2/1
  LKA_WhlBaseL_C=2.65/1 -> Switch2/3  "LKA_WhlBaseL_C"
  LKA_Veh2CamL_C=1.56/1 -> Switch1/3  "LKA_Veh2CamL_C"
  Data Type Conversion2/1 -> Switch1/2, Switch1/1
  Data Type Conversion13/1 -> Switch/2, Switch/1
  LKA_Veh2CamW_C=0.9/1 -> Switch/3  "LKA_Veh2CamW_C"

== system G59_LKAS_Carsim/LLClb/LDWClb ==
  Bus Creator : BusCreator  Inputs=1
  Data Type Conversion6 : DataTypeConversion  OutDataTypeStr=single
  LL_LDWS_SUPPRESS_HEADING=2 : Constant  Value=LL_LDWS_SUPPRESS_HEADING  OutDataTypeStr=single
  Switch2 : Switch  Criteria=u2 ~= 0  OutDataTypeStr=single
  LDWClb : Outport
  wires:
  Data Type Conversion6/1 -> Switch2/2, Switch2/1
  LL_LDWS_SUPPRESS_HEADING=2/1 -> Switch2/3
  Switch2/1 -> Bus Creator/1  "LL_LDWS_SUPPRESS_HEADING"
  Bus Creator/1 -> LDWClb/1
